simulink model "DC_Motor_Driver_Block_RPi"
settings: Solver=FixedStepDiscrete  StartTime=0.0  StopTime=inf  FixedStep=.1  RelTol=1e-3
PreSaveFcn:
  | set_param(gcs, 'location', [15 50 815 560])
settings Model: SimulationMode=external  ExtModeTrigDuration=100  Creator=The MathWorks Inc.  LastModifiedBy=hurstj
settings DataIOCC: LimitDataPoints=on  SaveFormat=Array  SignalLoggingSaveFormat=ModelDataLogs  ReturnWorkspaceOutputs=off
settings OptimizationCC: ExpressionDepthLimit=2147483647  OptimizeModelRefInitCode=on  LifeSpan=Inf  SimCompilerOptimization=Off
settings DebuggingCC: UnderspecifiedInitializationDetection=Classic  MergeDetectMultiDrivingBlocksExec=none  FcnCallInpInsideContextMsg=EnableAllAsWarning  FrameProcessingCompatibilityMsg=warning  StateNameClashWarn=warning  StrictBusMsg=Warning  SFUnexpectedBacktrackingDiag=warning  SFNoUnconditionalDefaultTransitionDiag=warning
settings HardwareCC: ProdBitPerPointer=32  ProdLargestAtomicInteger=Long  ProdLargestAtomicFloat=Double  ProdIntDivRoundTo=Undefined  ProdWordSize=32  ProdHWDeviceType=ARM Compatible->ARM Cortex
settings ModelReferenceCC: PropagateSignalLabelsOutOfModel=off
settings SFSimCC: SimUseLocalCustomCode=off
settings RTWCC: SystemTargetFile=realtime.tlc  GenerateMakefile=off  TemplateMakefile=realtime.tmf  Description=Run on Target Hardware  RTWVerbose=off  ProcessScript=realtime_make_rtw_hook  RTWUseLocalCustomCode=off  CustomInclude=/home/pi/wiringPi/wiringPi/  RTWCompilerOptimization=Off
settings CodeAppCC: CustomSymbolStrType=$N$R$M  InternalIdentifier=Classic
settings STFCustomTargetCC: TargetLibSuffix=.a  CodeReplacementLibrary=ANSI_C  GenerateSampleERTMain=on  ERTCustomFileBanners=on  SupportNonInlinedSFcns=off  SupportVariableSizeSignals=on  MATLABClassNameForMDSCustomization=Simulink.SoftwareTarget.ERTCustomization  GRTInterface=off  SystemTargetFile=realtime.tlc
settings ERTTargetCC: CodeReplacementLibrary=ANSI_C  MultiwordLength=2048  GenerateSampleERTMain=on  ParMdlRefBuildCompliant=off  CompOptLevelCompliant=off  ConcurrentExecutionCompliant=off  CombineOutputUpdateFcns=off  ERTFirstTimeCompliant=off  SupportContinuousTime=on  SupportVariableSizeSignals=on  ModelStepFunctionPrototypeControlCompliant=off  CPPClassGenCompliant=off  ExtMode=on  ExtModeMexArgs='192.168.2.13' 0 17725  InlinedParameterPlacement=NonHierarchical  ERTSrcFileBannerTemplate=realtime_code_template.cgt  ERTHdrFileBannerTemplate=realtime_code_template.cgt  ERTDataSrcFileTemplate=realtime_code_template.cgt  ERTDataHdrFileTemplate=realtime_code_template.cgt  ERTCustomFileTemplate=realtime_file_process.tlc  ConvertIfToSwitch=off  SuppressUnreachableDefaultCases=off

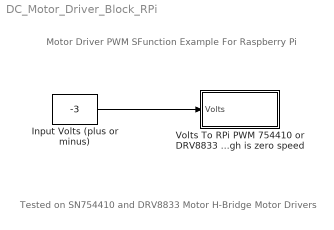
== system DC_Motor_Driver_Block_RPi ==
  note: Tested on SN754410 and DRV8833 Motor H-Bridge Motor Drivers
  note: Motor Driver PWM SFunction Example
      | For Raspberry Pi
  Input Volts (plus or minus) : Constant  Value=-3
  Volts To RPi PWM 754410 or DRV8833 PWM High is zero speed : Subsystem
  wires:
  Input Volts (plus or minus)/1 -> Volts To RPi PWM 754410 or DRV8833 PWM High is zero speed/1(Volts)

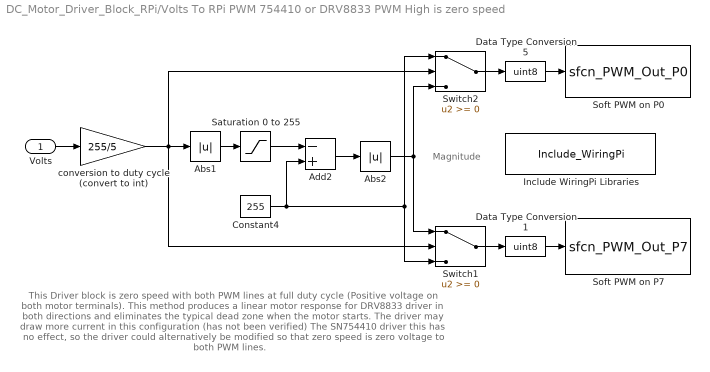
== system DC_Motor_Driver_Block_RPi/Volts To RPi PWM 754410 or DRV8833 PWM High is zero speed ==
  note: This Driver block is zero speed with both PWM lines at full duty cycle
      |  (Positive voltage on both motor terminals).
      | This method produces a linear motor response for DRV8833 driver
      |  in both directions and eliminates
      | the typical dead zone when the motor starts.
      | The driver may draw more current in this configuration (has not been verified)
      |
      | The SN754410 driver this has no effect, so the driver could alternatively
      | be modified so that zero speed is zero voltage to both PWM lines.
  note: Magnitude
  Volts : Inport
  Abs1 : Abs
  Abs2 : Abs
  Add2 : Sum  Inputs=-+
  Constant4 : Constant  Value=255
  Data Type Conversion1 : DataTypeConversion  OutDataTypeStr=uint8
  Data Type Conversion5 : DataTypeConversion  OutDataTypeStr=uint8
  Include WiringPi Libraries : S-Function  InitFcn=try, set_param(gcb,'FunctionName','Include_WiringPi'), end  FunctionName=Include_WiringPi  SFunctionModules=Include_WiringPi_wrapper  EnableBusSupport=off  mask(S-Function Builder){}
      mask help: Simulink:masks:SFunctionBuilder_MD
      mask init:
      | val = [[.9  0.75 0.75 1 1 .9 .9 1]',[1 1 0.75 0.75 .9 .9 1 .9]'];try , sys = get_param(gcb,'SfunBuilderFcnName');if isempty(sys), sys = get_param(gcb,'FunctionName'); end,catch, sys = get_param(gcb,'FunctionName'); end
      settings: CopyFcn=set_param(gcbh,'LinkStatus','none')  PreSaveFcn=try, set_param(gcb,'FunctionName','Include_WiringPi'), end  OpenFcn=sfunctionwizard(gcbh)
      mask Display:
      | plot(val(:,1),val(:,2))
      | disp(sys)
  Saturation 0 to 255 : Saturate  UpperLimit=255  LowerLimit=0
  Soft PWM on P0 : S-Function  InitFcn=try, set_param(gcb,'FunctionName','sfcn_PWM_Out_P0'), end  FunctionName=sfcn_PWM_Out_P0  Parameters=uint8(0)  SFunctionModules=sfcn_PWM_Out_P0_wrapper  EnableBusSupport=off  mask(S-Function Builder){}
      mask init: same as DC_Motor_Driver_Block_RPi/Volts To RPi PWM 754410 or DRV8833 PWM High is zero speed/Include WiringPi Libraries
      settings: CopyFcn=set_param(gcbh,'LinkStatus','none')  PreSaveFcn=try, set_param(gcb,'FunctionName','sfcn_PWM_Out_P0'), end  OpenFcn=sfunctionwizard(gcbh)
      mask Display: plot(val(:,1),val(:,2)),disp(sys), port_label('input',1,'in')
  Soft PWM on P7 : S-Function  InitFcn=try, set_param(gcb,'FunctionName','sfcn_PWM_Out_P7'), end  FunctionName=sfcn_PWM_Out_P7  Parameters=uint8(7)  SFunctionModules=sfcn_PWM_Out_P7_wrapper  EnableBusSupport=off  mask(S-Function Builder){}
      mask init: same as DC_Motor_Driver_Block_RPi/Volts To RPi PWM 754410 or DRV8833 PWM High is zero speed/Include WiringPi Libraries
      settings: CopyFcn=set_param(gcbh,'LinkStatus','none')  PreSaveFcn=try, set_param(gcb,'FunctionName','sfcn_PWM_Out_P7'), end  OpenFcn=sfunctionwizard(gcbh)
      mask Display: plot(val(:,1),val(:,2)),disp(sys), port_label('input',1,'in')
  Switch1 : Switch
  Switch2 : Switch
  conversion to duty cycle (convert to int) : Gain  Gain=255/5  OutDataTypeStr=int16
  wires:
  Volts/1 -> conversion to duty cycle (convert to int)/1
  conversion to duty cycle (convert to int)/1 -> Abs1/1, Switch2/2, Switch1/2
  Saturation 0 to 255/1 -> Add2/1
  Abs1/1 -> Saturation 0 to 255/1
  Constant4/1 -> Switch1/3, Switch2/1, Add2/2
  Add2/1 -> Abs2/1
  Abs2/1 -> Switch2/3, Switch1/1
  Switch2/1 -> Data Type Conversion5/1
  Switch1/1 -> Data Type Conversion1/1
  Data Type Conversion5/1 -> Soft PWM on P0/1
  Data Type Conversion1/1 -> Soft PWM on P7/1
